simulink model "version3"  (R2021a)
settings: Solver=VariableStepAuto  StartTime=0.0  StopTime=10.0  RelTol=1e-3
settings Model: Creator=Aashish Kalra  LastModifiedBy=Aashish Kalra
settings OptimizationCC: DefaultUnderspecifiedDataType=single
settings DebuggingCC: UniqueDataStoreMsg=error  StrictBusMsg=ErrorOnBusTreatedAsVector

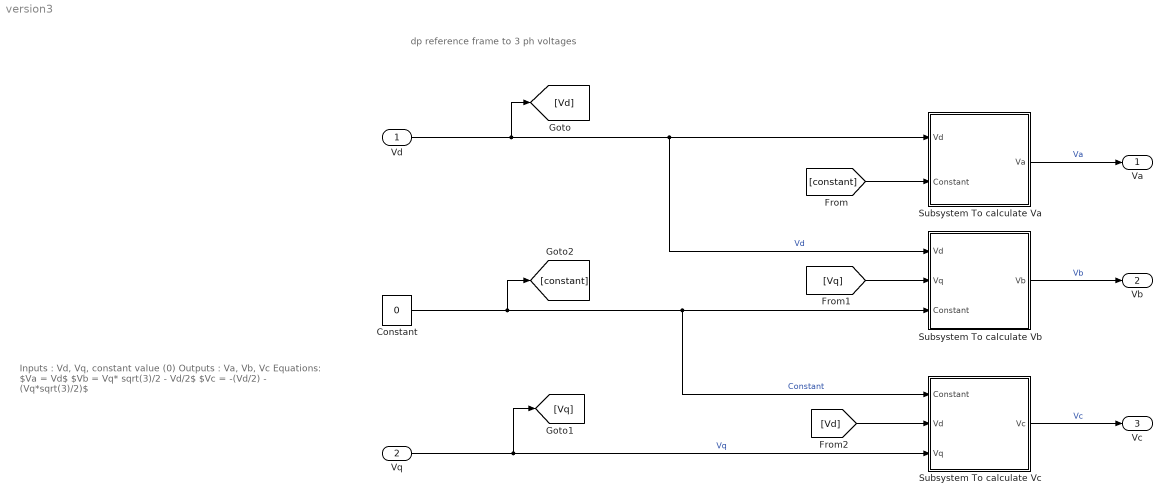
== system version3 ==
  note: Inputs : Vd, Vq, constant value (0)
      | Outputs : Va, Vb, Vc
      |
      | Equations:
      |
      | $Va = Vd$
      | $Vb = Vq* sqrt(3)/2 - Vd/2$
      | $Vc = -(Vd/2) - (Vq*sqrt(3)/2)$
  note: dp reference frame to 3 ph voltages
  Vd : Inport
  Vq : Inport  Port=2
  Constant : Constant  Value=0
  Subsystem To calculate Va : Subsystem
  Subsystem To calculate Vb : Subsystem
  Subsystem To calculate Vc : Subsystem
  Va : Outport  VectorParamsAs1DForOutWhenUnconnected=off
  Vb : Outport  Port=2  VectorParamsAs1DForOutWhenUnconnected=off
  Vc : Outport  Port=3  VectorParamsAs1DForOutWhenUnconnected=off
  wires:
  [Vd] -> Subsystem To calculate Vc/2(Vd)
  [constant] -> Subsystem To calculate Va/2(Constant)
  Subsystem To calculate Vb/1(Vb) -> Vb/1  "Vb"
  Vd/1 -> [Vd], Subsystem To calculate Vb/1(Vd), Subsystem To calculate Va/1(Vd)  "Vd"
  [Vq] -> Subsystem To calculate Vb/2(Vq)
  Constant/1 -> [constant], Subsystem To calculate Vc/1(Constant), Subsystem To calculate Vb/3(Constant)  "Constant"
  Vq/1 -> [Vq], Subsystem To calculate Vc/3(Vq)  "Vq"
  Subsystem To calculate Vc/1(Vc) -> Vc/1  "Vc"
  Subsystem To calculate Va/1(Va) -> Va/1  "Va"

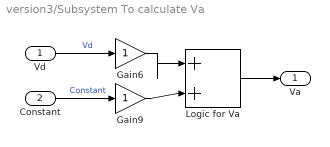
== system version3/Subsystem To calculate Va ==
  Vd : Inport
  Constant : Inport  Port=2
  Gain6 : Gain
  Gain9 : Gain
  Logic for Va : Sum  Inputs=|++
  Va : Outport
  wires:
  Vd/1 -> Gain6/1  "Vd"
  Constant/1 -> Gain9/1  "Constant"
  Gain6/1 -> Logic for Va/1
  Gain9/1 -> Logic for Va/2
  Logic for Va/1 -> Va/1

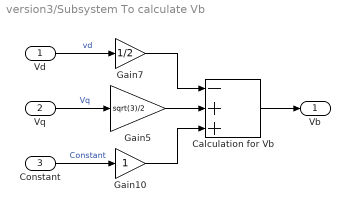
== system version3/Subsystem To calculate Vb ==
  Vd : Inport
  Vq : Inport  Port=2
  Constant : Inport  Port=3
  Calculation for Vb : Sum  Inputs=-++
  Gain10 : Gain
  Gain5 : Gain  Gain=sqrt(3)/2
  Gain7 : Gain  Gain=1/2
  Vb : Outport
  wires:
  Vq/1 -> Gain5/1  "Vq"
  Vd/1 -> Gain7/1  "vd"
  Constant/1 -> Gain10/1  "Constant"
  Gain7/1 -> Calculation for Vb/1
  Calculation for Vb/1 -> Vb/1
  Gain10/1 -> Calculation for Vb/3
  Gain5/1 -> Calculation for Vb/2

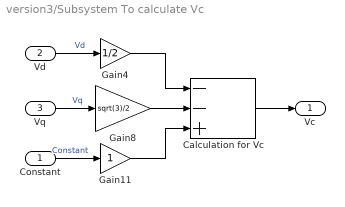
== system version3/Subsystem To calculate Vc ==
  Constant : Inport
  Vd : Inport  Port=2
  Vq : Inport  Port=3
  Calculation for Vc : Sum  Inputs=--+
  Gain11 : Gain
  Gain4 : Gain  Gain=1/2
  Gain8 : Gain  Gain=sqrt(3)/2
  Vc : Outport
  wires:
  Constant/1 -> Gain11/1  "Constant"
  Gain11/1 -> Calculation for Vc/3
  Calculation for Vc/1 -> Vc/1
  Vd/1 -> Gain4/1  "Vd"
  Gain4/1 -> Calculation for Vc/1
  Gain8/1 -> Calculation for Vc/2
  Vq/1 -> Gain8/1  "Vq"
